simulink model "threelevel_12phase1"  (R2020b)
settings: Solver=FixedStepDiscrete  StartTime=0.0  StopTime=1  FixedStep=Ts_FEA  RelTol=1e-3
model workspace (MAT data in the model file):
  T_10kHz = Simulink.Parameter
  T_10kHz.DataType = 'auto'
  T_10kHz.Dimensions = [0 0]
undefined symbols (not defined in the file): Cin, DiscIntNeverNeededParam, ESL, ESR, faif, Jm, kfeed_r, ki_n, kp_n, L, Ld, Line, Lq, ncmd_climb, ncmd_cruise, ncmd_run, ncmd_takeoff, p, Pcmd_climb, Pcmd_cruise, Pcmd_run, Pcmd_takeoff, Rs, Tcmd_run, Tcmd_start, Tcmd_time, time_climb, time_cruise, time_run, time_start, time_takeoff, Ts, Ts_Dead, Ts_FEA, Ts_speedloop, tswitch_climb, tswitch_takeoff, VDC, ws, zero_C1
libraries: powerlib x73, simulink x16, powerlib_meascontrol x16, slpidlib x13
(part 1 of 6)
settings Model: SimulationMode=accelerator  Creator=Shaoy  LastModifiedBy=HP
settings SolverCC: MinimalZcImpactIntegration=on
settings DataIOCC: InitialState=xIntial  LoadInitialState=on  SaveFinalState=on  SaveOperatingPoint=on  SaveOutput=off  SignalLogging=off  DSMLogging=off  SaveTime=off  ReturnWorkspaceOutputs=off
settings DebuggingCC: ReadBeforeWriteMsg=DisableAll  WriteAfterWriteMsg=DisableAll  WriteAfterReadMsg=DisableAll  MultiTaskDSMMsg=none
settings ModelReferenceCC: UpdateModelReferenceTargets=IfOutOfDate
settings SFSimCC: SFSimEcho=off

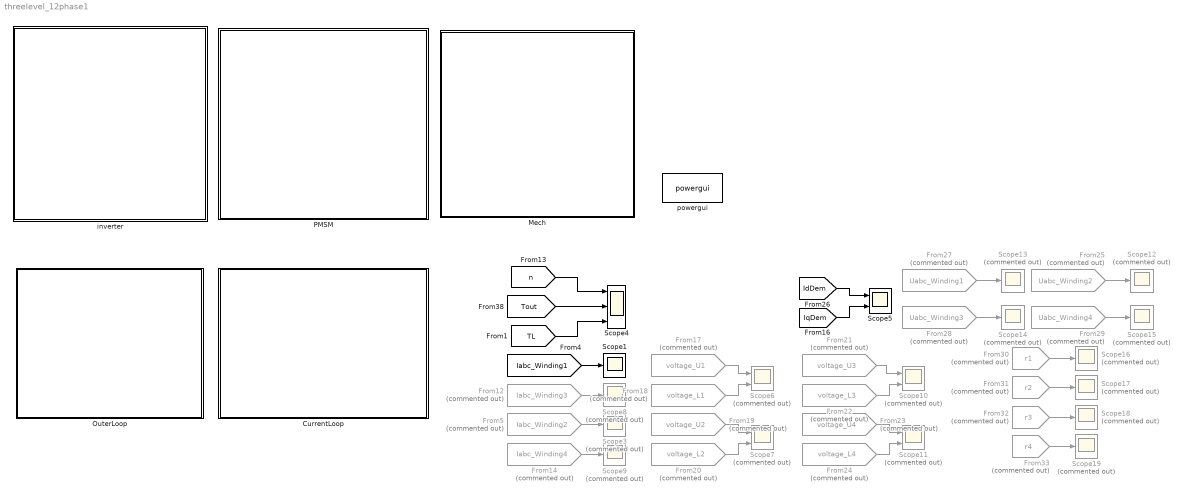
== system threelevel_12phase1 ==
  CurrentLoop : Subsystem
  From12 : From  Commented=on  GotoTag=Iabc_Winding3  TagVisibility=global
  From14 : From  Commented=on  GotoTag=Iabc_Winding4  TagVisibility=global
  From17 : From  Commented=on  GotoTag=voltage_U1  TagVisibility=global
  From18 : From  Commented=on  GotoTag=voltage_L1  TagVisibility=global
  From19 : From  Commented=on  GotoTag=voltage_U2  TagVisibility=global
  From20 : From  Commented=on  GotoTag=voltage_L2  TagVisibility=global
  From21 : From  Commented=on  GotoTag=voltage_U3  TagVisibility=global
  From22 : From  Commented=on  GotoTag=voltage_L3  TagVisibility=global
  From23 : From  Commented=on  GotoTag=voltage_U4  TagVisibility=global
  From24 : From  Commented=on  GotoTag=voltage_L4  TagVisibility=global
  From25 : From  Commented=on  GotoTag=Uabc_Winding2  TagVisibility=global
  From27 : From  Commented=on  GotoTag=Uabc_Winding1  TagVisibility=global
  From28 : From  Commented=on  GotoTag=Uabc_Winding3  TagVisibility=global
  From29 : From  Commented=on  GotoTag=Uabc_Winding4  TagVisibility=global
  From30 : From  Commented=on  GotoTag=r1  TagVisibility=global
  From31 : From  Commented=on  GotoTag=r2  TagVisibility=global
  From32 : From  Commented=on  GotoTag=r3  TagVisibility=global
  From33 : From  Commented=on  GotoTag=r4  TagVisibility=global
  From5 : From  Commented=on  GotoTag=Iabc_Winding2  TagVisibility=global
  Mech : Subsystem
  OuterLoop : Subsystem
  PMSM : Subsystem
  Scope1 : Scope
  Scope{6..7,10..11} (4 alike) : Scope  Commented=on  NumInputPorts=2
  Scope{3,8..9,12..19} (11 alike) : Scope  Commented=on
  Scope4 : Scope  NumInputPorts=3
  Scope5 : Scope  NumInputPorts=2
  inverter : Subsystem
  powergui : powerlib/powergui  Priority=1  SimulationMode=Discrete  SampleTime=Ts_FEA  frequency=60  Iterations=50  frequencyindice=0  Pbase=100e6  ErrMax=1e-4  UnitsV=kV  UnitsW=MW  buscounter=0  FunctionMessages=off  echomessages=off  EnableUseOfTLC=off  CurrentSourceSwitches=off  DisableSnubberDevices=off  DisableRonSwitches=off  DisableVfSwitches=off  DisplayEquations=off  AutomaticDiscreteSolvers=off  SolverType=Tustin/Backward Euler (TBE)  Interpol=off  ExternalGateDelay=off  methode=off  Ts=100  x0status=blocks  SPID=on  SwTol=0  HookPort=off  NonlinearTolerance=1e-4  nMaxIteration=100  ContinueOnMaxIteration=off  RestoreLinks=warning  ResistiveCurrentMeasurement=off  Frange=[0:2:500]  Ylog=off  Xlog=on  ShowGrid=off  save=off  variable=ZData  structure=Mech_out  ZoomFFT=off  StartTime=0.63  cycles=1  DisplayStyle=4  fundamental=6997*4/60  FreqAxis=off  MaxFrequency=100000  frequencyindicesteady=1  RmsSteady=1  display=off
  wires:
  [Iabc_Winding1] -> Scope1/1
  From5/1 -> Scope3/1
  From12/1 -> Scope8/1
  From14/1 -> Scope9/1
  [IqDem] -> Scope5/2
  From17/1 -> Scope6/1
  From18/1 -> Scope6/2
  From19/1 -> Scope7/1
  From20/1 -> Scope7/2
  From21/1 -> Scope10/1
  From22/1 -> Scope10/2
  From23/1 -> Scope11/1
  From24/1 -> Scope11/2
  From25/1 -> Scope12/1
  [IdDem] -> Scope5/1
  From27/1 -> Scope13/1
  From28/1 -> Scope14/1
  From29/1 -> Scope15/1
  From30/1 -> Scope16/1
  From31/1 -> Scope17/1
  From32/1 -> Scope18/1
  From33/1 -> Scope19/1
  [n] -> Scope4/1
  [Tout] -> Scope4/2
  [TL] -> Scope4/3

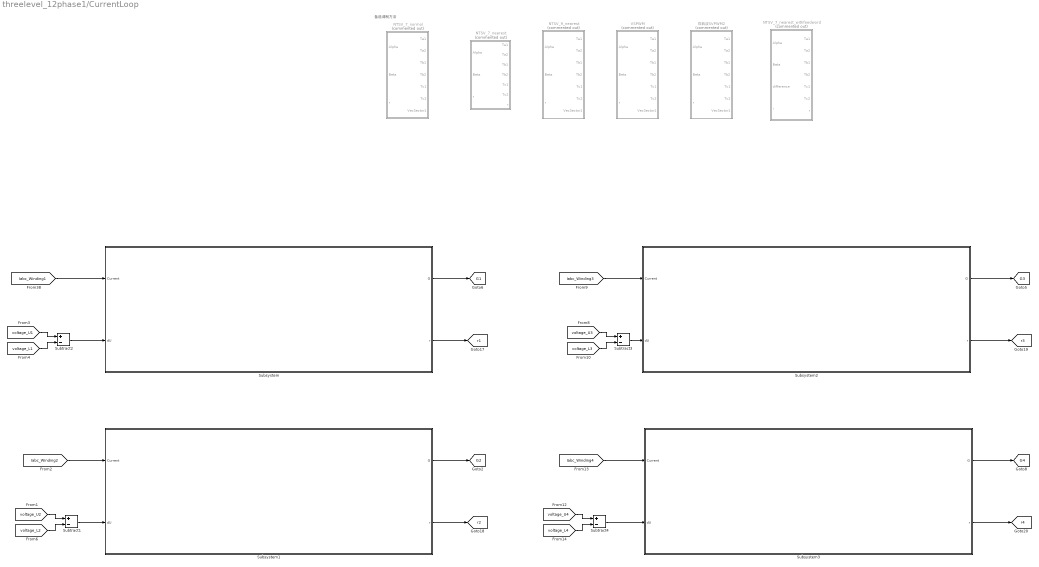
== system threelevel_12phase1/CurrentLoop ==
  note: 备选调制方法
  NTSV_7_nearest : MATLAB Function  Commented=on  TreatAsAtomicUnit=on
  NTSV_7_nearest_withfeedword : MATLAB Function  Commented=on  TreatAsAtomicUnit=on
  NTSV_7_normol : MATLAB Function  Commented=on  TreatAsAtomicUnit=on
  NTSV_9_nearest : MATLAB Function  Commented=on  TreatAsAtomicUnit=on
  Subsystem : Subsystem
  Subsystem1 : Subsystem
  Subsystem2 : Subsystem
  Subsystem3 : Subsystem
  Subtract{1..4} (4 alike) : Sum  Inputs=+-
  VSPWM : MATLAB Function  Commented=on  TreatAsAtomicUnit=on
  双载波SVPWM2 : MATLAB Function  Commented=on  TreatAsAtomicUnit=on
  tag scope: G1=global, G2=global, G3=global, G4=global, r1=global, r2=global, r3=global, r4=global
  wires:
  [voltage_U1] -> Subtract2/1
  [voltage_L1] -> Subtract2/2
  [voltage_L3] -> Subtract3/2
  [voltage_U3] -> Subtract3/1
  [voltage_L4] -> Subtract4/2
  [voltage_U4] -> Subtract4/1
  Subtract2/1 -> Subsystem/2(dU)
  [Iabc_Winding1] -> Subsystem/1(Current)
  Subsystem/2(r) -> [r1]
  Subsystem/1(G) -> [G1]
  Subtract1/1 -> Subsystem1/2(dU)
  [voltage_L2] -> Subtract1/2
  [voltage_U2] -> Subtract1/1
  [Iabc_Winding2] -> Subsystem1/1(Current)
  Subsystem1/2(r) -> [r2]
  Subsystem1/1(G) -> [G2]
  [Iabc_Winding3] -> Subsystem2/1(Current)
  Subtract3/1 -> Subsystem2/2(dU)
  Subsystem2/2(r) -> [r3]
  Subsystem2/1(G) -> [G3]
  Subsystem3/1(G) -> [G4]
  Subsystem3/2(r) -> [r4]
  [Iabc_Winding4] -> Subsystem3/1(Current)
  Subtract4/1 -> Subsystem3/2(dU)

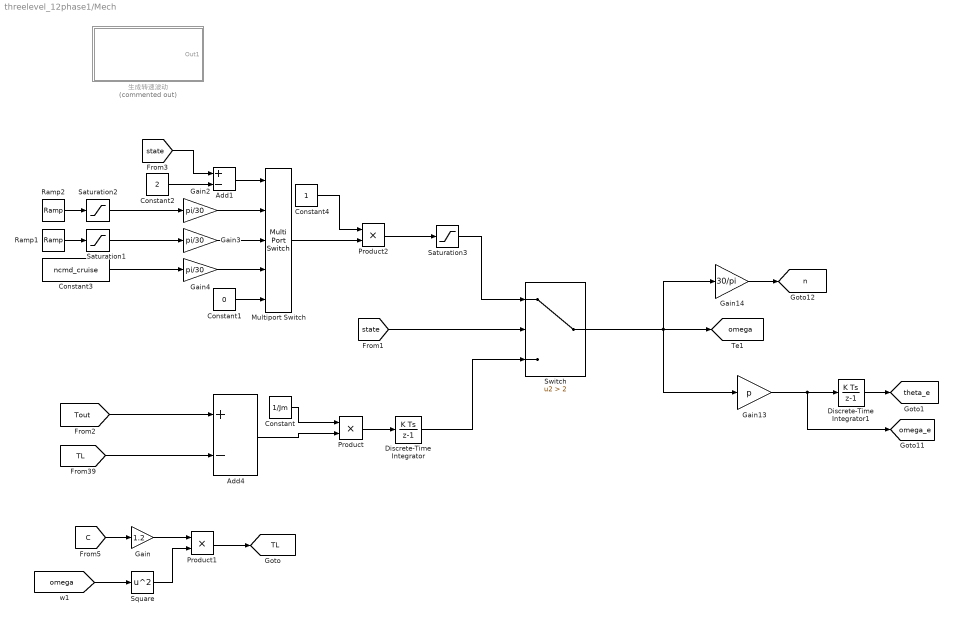
== system threelevel_12phase1/Mech ==
  Add1 : Sum  Inputs=+-
  Add4 : Sum  Inputs=+-
  Constant : Constant  Value=1/Jm  SampleTime=-1
  Constant1 : Constant  Value=0
  Constant2 : Constant  Value=2
  Constant3 : Constant  Value=ncmd_cruise
  Constant4 : Constant
  Discrete-Time Integrator : DiscreteIntegrator  SampleTime=-1  ICPrevOutput=DiscIntNeverNeededParam  ICPrevScaledInput=DiscIntNeverNeededParam
  Discrete-Time Integrator1 : DiscreteIntegrator  SampleTime=-1  ICPrevOutput=DiscIntNeverNeededParam  ICPrevScaledInput=DiscIntNeverNeededParam
  Gain : Gain  Gain=1.2
  Gain13 : Gain  Gain=p
  Gain14 : Gain  Gain=30/pi
  Gain2 : Gain  Gain=pi/30
  Gain3 : Gain  Gain=pi/30
  Gain4 : Gain  Gain=pi/30
  Multiport Switch : MultiPortSwitch  DataPortForDefault=Additional data port  DiagnosticForDefault=None
  Product : Product
  Product1 : Product
  Product2 : Product
  Ramp1 : simulink/Sources/Ramp  slope=(ncmd_climb-ncmd_takeoff)/tswitch_climb  start=time_takeoff  InitialOutput=ncmd_takeoff
  Ramp2 : simulink/Sources/Ramp  slope=(ncmd_takeoff-ncmd_run)/tswitch_takeoff  start=time_run  InitialOutput=ncmd_run
  Saturation1 : Saturate  UpperLimit=ncmd_takeoff  LowerLimit=ncmd_climb
  Saturation2 : Saturate  UpperLimit=ncmd_takeoff  LowerLimit=ncmd_run
  Saturation3 : Saturate  UpperLimit=988  LowerLimit=0
  Square : Math  Operator=square  SaturateOnIntegerOverflow=on
  Switch : Switch  Criteria=u2 > Threshold  Threshold=2
  生成转速波动 : Subsystem  Commented=on
  tag scope: TL=global, n=global, omega=global, omega_e=global, theta_e=global
  wires:
  [Tout] -> Add4/1
  Add4/1 -> Product/2
  Product/1 -> Discrete-Time Integrator/1
  Constant/1 -> Product/1
  [TL] -> Add4/2
  Gain14/1 -> [n]
  [C] -> Gain/1
  Gain/1 -> Product1/1
  Product1/1 -> [TL]
  [omega] -> Square/1
  Square/1 -> Product1/2
  Discrete-Time Integrator1/1 -> [theta_e]
  Gain13/1 -> [omega_e], Discrete-Time Integrator1/1
  Switch/1 -> Gain14/1, Gain13/1, [omega]
  [state] -> Switch/2
  Discrete-Time Integrator/1 -> Switch/3
  Constant1/1 -> Multiport Switch/5
  [state] -> Add1/1
  Add1/1 -> Multiport Switch/1
  Constant2/1 -> Add1/2
  Gain4/1 -> Multiport Switch/4
  Gain3/1 -> Multiport Switch/3
  Gain2/1 -> Multiport Switch/2
  Saturation2/1 -> Gain2/1
  Saturation1/1 -> Gain3/1
  Constant3/1 -> Gain4/1
  Ramp2/1 -> Saturation2/1
  Ramp1/1 -> Saturation1/1
  Multiport Switch/1 -> Product2/2
  Product2/1 -> Saturation3/1
  Saturation3/1 -> Switch/1
  Constant4/1 -> Product2/1

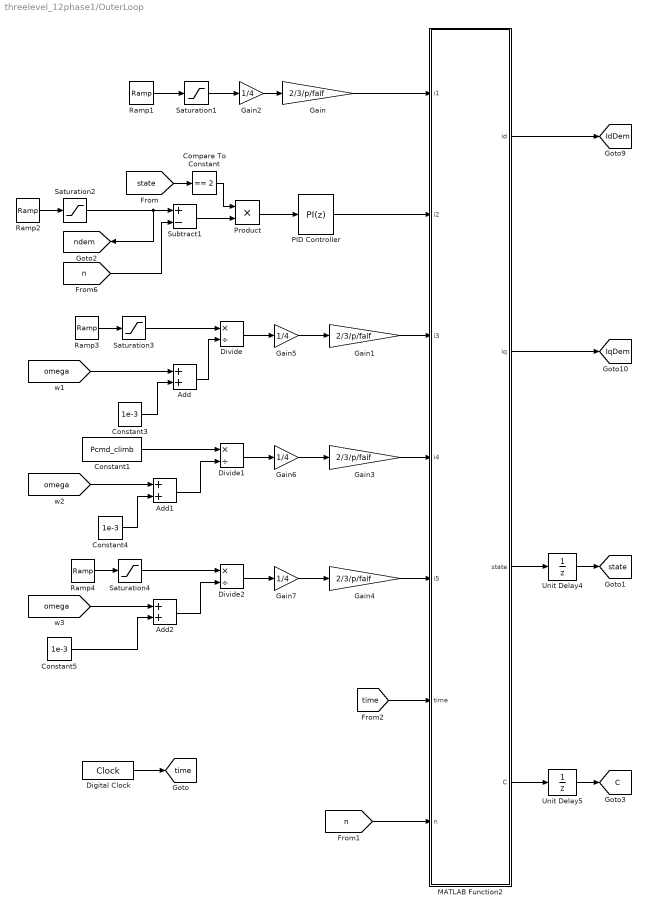
== system threelevel_12phase1/OuterLoop ==
  Add : Sum
  Add1 : Sum
  Add2 : Sum
  Compare To Constant : simulink/Logic and Bit Operations/Compare To Constant  relop===  const=2  OutDataTypeStr=boolean
  Constant1 : Constant  Value=Pcmd_climb
  Constant3 : Constant  Value=1e-3
  Constant4 : Constant  Value=1e-3
  Constant5 : Constant  Value=1e-3
  Digital Clock : DigitalClock
  Divide : Product  Inputs=*/
  Divide1 : Product  Inputs=*/
  Divide2 : Product  Inputs=*/
  Gain{,1,3..4} (4 alike) : Gain  Gain=2/3/p/faif
  Gain{2,5..7} (4 alike) : Gain  Gain=1/4
  MATLAB Function2 : MATLAB Function  TreatAsAtomicUnit=on
  PID Controller : slpidlib/PID Controller  Controller=PI  Form=Parallel  TimeDomain=Discrete-time  UseExternalTs=off  SampleTime=Ts_speedloop  IntegratorMethod=Forward Euler  FilterMethod=Forward Euler  ControllerParametersSource=internal  P=kp_n  I=ki_n  D=0  UseFilter=on  N=100  TunerSelectOption=Transfer Function Based (PID Tuner App)  InitialConditionSource=internal  InitialConditionForIntegrator=2*Tcmd_run/4/3/p/faif  InitialConditionForFilter=0  DifferentiatorICPrevScaledInput=0  ExternalReset=none  TrackingMode=off  Kt=1  LimitOutput=off  SatLimitsSource=internal  UpperSaturationLimit=1  LowerSaturationLimit=-1  LinearizeAsGain=off  AntiWindupMode=none  Kb=1  POutMin=[]  POutMax=[]  IOutMin=[]  IOutMax=[]  DOutMin=[]  DOutMax=[]  NOutMin=[]  NOutMax=[]  SumOutMin=[]  SumOutMax=[]  SaturationOutMin=[]  SaturationOutMax=[]  PParamMin=[]  PParamMax=[]  IParamMin=[]  IParamMax=[]  DParamMin=[]  DParamMax=[]  NParamMin=[]  NParamMax=[]  KbParamMin=[]  KbParamMax=[]  KtParamMin=[]  KtParamMax=[]  KbOutMin=[]  KbOutMax=[]  KtOutMin=[]  KtOutMax=[]  IntegratorOutMin=[]  IntegratorOutMax=[]  FilterOutMin=[]  FilterOutMax=[]  SumI1OutMin=[]  SumI1OutMax=[]  SumI2OutMin=[]  SumI2OutMax=[]  SumI3OutMin=[]  SumI3OutMax=[]  SumI4OutMin=[]  SumI4OutMax=[]  SumDOutMin=[]  SumDOutMax=[]  DifferentiatorOutMin=[]  DifferentiatorOutMax=[]  FilterDiffOutCoefMin=[]  FilterDiffOutCoefMax=[]  ReciprocalOutMin=[]  ReciprocalOutMax=[]  SumDenOutMin=[]  SumDenOutMax=[]  SumNumOutMin=[]  SumNumOutMax=[]  DivideOutMin=[]  DivideOutMax=[]  UdiffTsProdOutMin=[]  UdiffTsProdOutMax=[]  NTsProdOutMin=[]  NTsProdOutMax=[]  UintegralTsProdOutMin=[]  UintegralTsProdOutMax=[]  UngainTsProdOutMin=[]  UngainTsProdOutMax=[]  IntegratorContinuousStateAttributes=''  IntegratorStateMustResolveToSignalObject=off  IntegratorRTWStateStorageClass=Auto  FilterContinuousStateAttributes=''  FilterStateMustResolveToSignalObject=off  FilterRTWStateStorageClass=Auto  ParallelPVariant=InternalParameters  IdealPVariant=Disabled  IVariant=InternalParameters  DVariant=Disabled  IntegratorVariant=Discrete  SatVariant=Disabled  AWVariant=Passthrough  PCopyVariant=Disabled  TRVariant=Disabled  FdbkBlocksVariant=Forward  IdealPFdbkVariant=Disabled  SatFdbkVariant=Disabled  DerivativeFilterVariant=Disabled  NVariant=Disabled  NCopyVariant=Disabled_SignalSpec  FilterICVariant=Disabled  IntegratorICVariant=InternalICs  ExternalResetVariant=Disabled  TRSumVariant=Passthrough  SumFdbkVariant=Disabled  SumVariant=Sum_PI  TsampFilterVariant=InternalTs  TsampNgainVariant=Passthrough  TsampIntegralVariant=Passthrough  ExternalSaturationOutDataTypeStr=Inherit: Same as second input
  Product : Product
  Ramp1 : simulink/Sources/Ramp  slope=Tcmd_start/Tcmd_time  start=0  InitialOutput=0
  Ramp2 : simulink/Sources/Ramp  slope=ncmd_run/0.1  start=0  InitialOutput=0
  Ramp3 : simulink/Sources/Ramp  slope=(Pcmd_takeoff-Pcmd_run)/tswitch_climb  start=time_run  InitialOutput=Pcmd_run
  Ramp4 : simulink/Sources/Ramp  slope=(Pcmd_cruise-Pcmd_climb)/tswitch_climb  start=time_climb  InitialOutput=Pcmd_climb
  Saturation1 : Saturate  UpperLimit=Tcmd_start  LowerLimit=0
  Saturation2 : Saturate  UpperLimit=ncmd_run  LowerLimit=0
  Saturation3 : Saturate  UpperLimit=Pcmd_takeoff  LowerLimit=0
  Saturation4 : Saturate  UpperLimit=Pcmd_takeoff  LowerLimit=Pcmd_cruise
  Subtract1 : Sum  Inputs=+-
  Unit Delay4 : UnitDelay  SampleTime=-1  HasFrameUpgradeWarning=on
  Unit Delay5 : UnitDelay  SampleTime=-1  HasFrameUpgradeWarning=on
  tag scope: C=global, IdDem=global, IqDem=global, ndem=global, state=global, time=global
  wires:
  Saturation1/1 -> Gain2/1
  Ramp1/1 -> Saturation1/1
  Gain2/1 -> Gain/1
  Saturation2/1 -> [ndem], Subtract1/1
  Ramp2/1 -> Saturation2/1
  Subtract1/1 -> Product/2
  Product/1 -> PID Controller/1
  Gain/1 -> MATLAB Function2/1(i1)
  PID Controller/1 -> MATLAB Function2/2(i2)
  Gain1/1 -> MATLAB Function2/3(i3)
  Add1/1 -> Divide1/2
  Constant1/1 -> Divide1/1
  Saturation4/1 -> Divide2/1
  Add2/1 -> Divide2/2
  MATLAB Function2/3(state) -> Unit Delay4/1
  MATLAB Function2/4(C) -> Unit Delay5/1
  [state] -> Compare To Constant/1
  Compare To Constant/1 -> Product/1
  MATLAB Function2/1(id) -> [IdDem]
  MATLAB Function2/2(iq) -> [IqDem]
  Constant3/1 -> Add/2
  Add/1 -> Divide/2
  Constant4/1 -> Add1/2
  Constant5/1 -> Add2/2
  Gain3/1 -> MATLAB Function2/4(i4)
  Gain4/1 -> MATLAB Function2/5(i5)
  [n] -> MATLAB Function2/7(n)
  [omega] -> Add/1
  [omega] -> Add1/1
  [omega] -> Add2/1
  Ramp3/1 -> Saturation3/1
  Saturation3/1 -> Divide/1
  Gain7/1 -> Gain4/1
  Divide2/1 -> Gain7/1
  Divide1/1 -> Gain6/1
  Gain6/1 -> Gain3/1
  Gain5/1 -> Gain1/1
  Divide/1 -> Gain5/1
  [n] -> Subtract1/2
  Unit Delay4/1 -> [state]
  Unit Delay5/1 -> [C]
  Ramp4/1 -> Saturation4/1
  [time] -> MATLAB Function2/6(time)
  Digital Clock/1 -> [time]

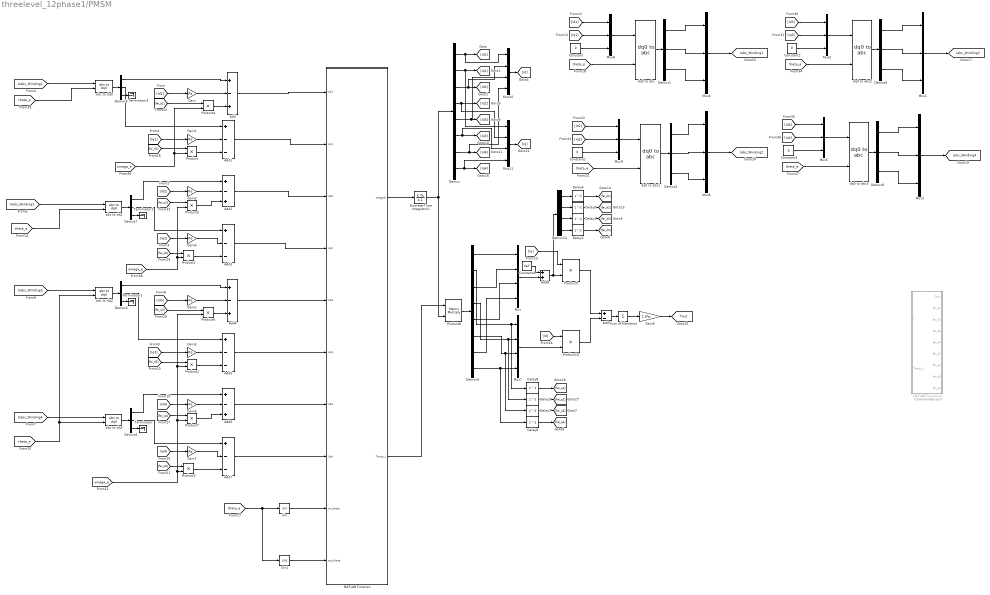
== system threelevel_12phase1/PMSM ==
  Add{,2,4,6} (4 alike) : Sum  Inputs=+-+
  Add{1,3,5,7} (4 alike) : Sum  Inputs=+--
  Add8 : Sum
  Add9 : Sum  Inputs=+-
  Constant{,1..3} (4 alike) : Constant  Value=0  SampleTime=-1
  Constant4 : Constant  Value=faif
  Delay{1..6,8..9} (8 alike) : Delay  DelayLength=1
  Demux : Demux  Outputs=8
  Demux{1..8} (8 alike) : Demux  Outputs=3
  Demux10 : Demux
  Demux9 : Demux  Outputs=8
  Discrete-Time Integrator1 : DiscreteIntegrator  SampleTime=-1  ICPrevOutput=DiscIntNeverNeededParam  ICPrevScaledInput=DiscIntNeverNeededParam
  Gain{,1..7} (8 alike) : Gain  Gain=Rs
  Gain8 : Gain  Gain=1.5*p
  MATLAB Function : MATLAB Function  TreatAsAtomicUnit=on
  MATLAB Function2 : MATLAB Function  Commented=on  TreatAsAtomicUnit=on
  Mux{,7,10..11} (4 alike) : Mux
  Mux{1..6,8..9} (8 alike) : Mux  Inputs=3
  Product{,1..7,9..10} (10 alike) : Product
  Product8 : Product  Multiplication=Matrix(*)
  Sin : Trigonometry
  Sin1 : Trigonometry  Operator=cos
  Sum of Elements : Sum  Inputs=+
  Terminator{,1..3} (4 alike) : Terminator
  abc to dq{0..3} (4 alike) : powerlib_meascontrol/Transformations/abc to dq0  Alignment=Aligned with phase A axis
  dq0 to abc{,1..3} (4 alike) : powerlib_meascontrol/Transformations/dq0 to abc  Alignment=Aligned with phase A axis
  tag scope: Iabc_Winding1=global, Iabc_Winding2=global, Iabc_Winding3=global, Iabc_Winding4=global, Tout=global
  wires:
  Demux5/2 -> Add1/1
  Demux5/1 -> Add/1
  Gain/1 -> Add/2
  [Id1] -> Gain/1
  [Iq1] -> Gain1/1
  Gain1/1 -> Add1/2
  Gain4/1 -> Add3/2
  [Iq2] -> Gain4/1
  [Id2] -> Gain3/1
  Gain3/1 -> Add2/2
  Demux7/1 -> Add2/1
  Demux7/2 -> Add3/1
  Add/1 -> MATLAB Function/1(Ud1)
  Add1/1 -> MATLAB Function/2(Uq1)
  [Uabc_Winding2] -> abc to dq1/1
  [Id1] -> Mux8/1
  [Iq1] -> Mux8/2
  Constant/1 -> Mux8/3
  [theta_e] -> abc to dq1/2
  [theta_e] -> dq0 to abc/2
  Demux1/1 -> Mux4/1
  Demux1/2 -> Mux4/2
  Demux1/3 -> Mux4/3
  Demux2/3 -> Mux6/3
  Demux2/2 -> Mux6/2
  Demux2/1 -> Mux6/1
  [theta_e] -> dq0 to abc1/2
  [Iq2] -> Mux9/2
  [Id2] -> Mux9/1
  Mux4/1 -> [Iabc_Winding1]
  Mux6/1 -> [Iabc_Winding2]
  Add2/1 -> MATLAB Function/3(Ud2)
  Add3/1 -> MATLAB Function/4(Uq2)
  abc to dq0/1 -> Demux5/1
  abc to dq1/1 -> Demux7/1
  Mux8/1 -> dq0 to abc/1
  dq0 to abc/1 -> Demux1/1
  dq0 to abc1/1 -> Demux2/1
  Mux9/1 -> dq0 to abc1/1
  Discrete-Time Integrator1/1 -> Product8/2, Demux/1
  [Uabc_Winding1] -> abc to dq0/1
  MATLAB Function/1(Integral) -> Discrete-Time Integrator1/1
  Demux/1 -> Mux10/1, [Id1]
  Demux/2 -> Mux11/1, [Iq1]
  Demux/3 -> Mux10/2, [Id2]
  Demux/4 -> Mux11/2, [Iq2]
  Constant1/1 -> Mux9/3
  Delay4/1 -> [fai_d1]
  Delay5/1 -> [fai_d2]
  Delay8/1 -> [fai_q1]
  Delay9/1 -> [fai_q2]
  Product/1 -> Add1/3
  [fai_d1] -> Product/1
  Product1/1 -> Add3/3
  [fai_d2] -> Product1/1
  Product4/1 -> Add/3
  [fai_q1] -> Product4/1
  Product5/1 -> Add2/3
  [fai_q2] -> Product5/1
  [Uabc_Winding4] -> abc to dq3/1
  [theta_e] -> abc to dq3/2, abc to dq2/2
  [Id3] -> Gain2/1
  Demux4/2 -> Add7/1
  Gain2/1 -> Add4/2
  Gain6/1 -> Add6/2
  [Iq4] -> Gain7/1
  Gain7/1 -> Add7/2
  Demux3/1 -> Add4/1
  [omega_e] -> Product7/2, Product6/2, Product2/2, Product3/2
  [Iq3] -> Gain5/1
  [fai_d3] -> Product2/1
  Demux4/1 -> Add6/1
  Product6/1 -> Add4/3
  Product7/1 -> Add6/3
  [fai_d4] -> Product3/1
  [fai_q4] -> Product7/1
  Product3/1 -> Add7/3
  Gain5/1 -> Add5/2
  Product2/1 -> Add5/3
  Demux3/2 -> Add5/1
  [Id4] -> Gain6/1
  [Uabc_Winding3] -> abc to dq2/1
  abc to dq2/1 -> Demux3/1
  [fai_q3] -> Product6/1
  abc to dq3/1 -> Demux4/1
  Add4/1 -> MATLAB Function/5(Ud3)
  Add5/1 -> MATLAB Function/6(Uq3)
  Add6/1 -> MATLAB Function/7(Ud4)
  Add7/1 -> MATLAB Function/8(Uq4)
  Delay1/1 -> [fai_d3]
  Delay2/1 -> [fai_d4]
  Delay6/1 -> [fai_q4]
  Delay3/1 -> [fai_q3]
  Demux/5 -> Mux10/3, [Id3]
  Demux/6 -> Mux11/3, [Iq3]
  Demux/7 -> Mux10/4, [Id4]
  Demux/8 -> Mux11/4, [Iq4]
  Mux1/1 -> [Iabc_Winding3]
  Mux2/1 -> dq0 to abc2/1
  Demux6/2 -> Mux1/2
  Constant2/1 -> Mux2/3
  dq0 to abc2/1 -> Demux6/1
  [Id3] -> Mux2/1
  [theta_e] -> dq0 to abc2/2
  Demux6/3 -> Mux1/3
  Demux6/1 -> Mux1/1
  [Iq3] -> Mux2/2
  Mux3/1 -> [Iabc_Winding4]
  Demux8/2 -> Mux3/2
  dq0 to abc3/1 -> Demux8/1
  Constant3/1 -> Mux5/3
  [theta_e] -> dq0 to abc3/2
  [Id4] -> Mux5/1
  [Iq4] -> Mux5/2
  Mux5/1 -> dq0 to abc3/1
  Demux8/3 -> Mux3/3
  Demux8/1 -> Mux3/1
  Demux4/3 -> Terminator/1
  Demux3/3 -> Terminator1/1
  Demux7/3 -> Terminator2/1
  Demux5/3 -> Terminator3/1
  [theta_e] -> Sin1/1, Sin/1
  Sin/1 -> MATLAB Function/9(sin_theta)
  Sin1/1 -> MATLAB Function/10(cos_theta)
  MATLAB Function/2(Temp_L) -> Product8/1
  Product8/1 -> Demux9/1
  Demux9/1 -> Mux/1
  Demux9/3 -> Mux/2
  Demux9/5 -> Mux/3
  Demux9/7 -> Mux/4
  Mux/1 -> Add8/2
  Constant4/1 -> Add8/1
  Demux9/8 -> Delay6/1, Mux7/4
  Demux9/6 -> Mux7/3, Delay3/1
  Demux9/2 -> Delay8/1, Mux7/1
  Demux9/4 -> Delay9/1, Mux7/2
  Mux10/1 -> [Id]
  Mux11/1 -> [Iq]
  Add8/1 -> Demux10/1, Product9/2
  [Iq] -> Product9/1
  Mux7/1 -> Product10/2
  [Id] -> Product10/1
  Product9/1 -> Add9/1
  Product10/1 -> Add9/2
  Add9/1 -> Sum of Elements/1
  Sum of Elements/1 -> Gain8/1
  Gain8/1 -> [Tout]
  Demux10/1 -> Delay4/1
  Demux10/2 -> Delay5/1
  Demux10/3 -> Delay1/1
  Demux10/4 -> Delay2/1
  [theta_e] -> abc to dq0/2
  [omega_e] -> Product5/2, Product1/2
  [omega_e] -> Product4/2, Product/2

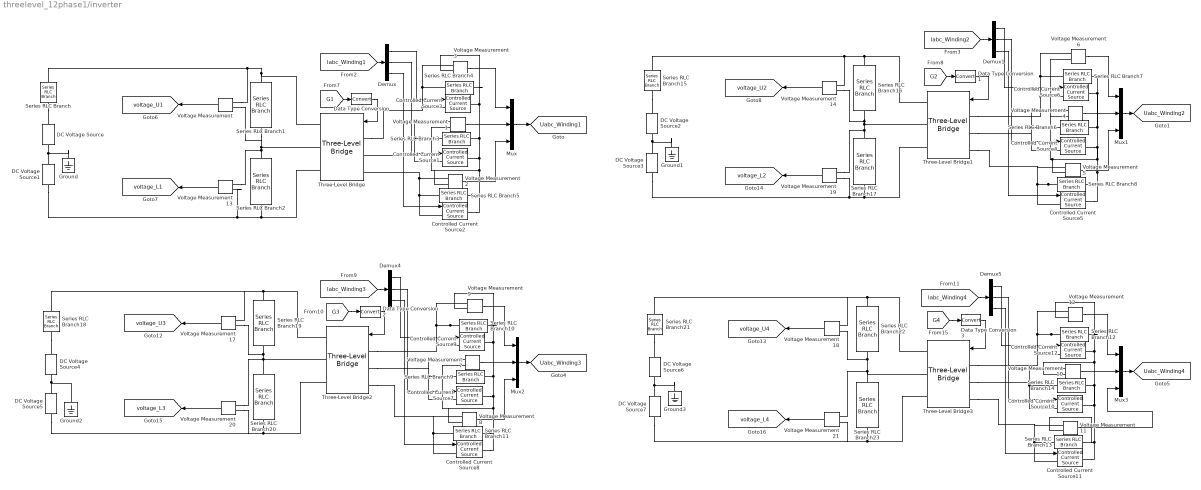
== system threelevel_12phase1/inverter ==
  Controlled Current Source{1..12} (12 alike) : powerlib/Electrical Sources/Controlled Current Source  Initialize=on  Source_Type=AC  Amplitude=0  Phase=0  Frequency=0  Measurements=None
  DC Voltage Source{,1..7} (8 alike) : powerlib/Electrical Sources/DC Voltage Source  Amplitude=VDC/2  Measurements=None
  Data Type Conversion{,1..3} (4 alike) : DataTypeConversion
  Demux{,1,4..5} (4 alike) : Demux  Outputs=3
  Ground{,1..3} (4 alike) : powerlib/Elements/Ground  LConnTagsString=a
  Mux{,1..3} (4 alike) : Mux  Inputs=3
  Series RLC Branch{,15,18,21} (4 alike) : powerlib/Elements/Series RLC Branch  LConnTagsString=__new0  RConnTagsString=__new0  BranchType=L  Resistance=1  Inductance=Line  SetiL0=off  InitialCurrent=0  Capacitance=1e-6  Setx0=off  InitialVoltage=0  Measurements=None
  Series RLC Branch{1..2,16..17,19..20,22..23} (8 alike) : powerlib/Elements/Series RLC Branch  LConnTagsString=__new0  RConnTagsString=__new0  BranchType=RLC  Resistance=ESR  Inductance=ESL  SetiL0=off  InitialCurrent=0  Capacitance=Cin  Setx0=off  InitialVoltage=0  Measurements=None
  Series RLC Branch{3..14} (12 alike) : powerlib/Elements/Series RLC Branch  LConnTagsString=__new0  RConnTagsString=__new0  BranchType=R  Resistance=10^6  Inductance=51.869e-9  SetiL0=off  InitialCurrent=0  Capacitance=330e-6  Setx0=off  InitialVoltage=0  Measurements=None
  Three-Level Bridge{,1..3} (4 alike) : powerlib/Power Electronics/Three-Level Bridge  Arms=3  SnubberResistance=1e5  SbubberCapacitance=inf  Device=IGBT / Diodes  Ron=3.1e-3  ForwardVoltages="[  0.77  0.9  ]"  Measurements=None
      settings: SourceProductBaseCode=PS
  Voltage Measurement{,1..14,17..21} (20 alike) : powerlib/Measurements/Voltage Measurement  PhasorSimulation=off  OutputType=Complex  PSBequivalent=0
  tag scope: Uabc_Winding1=global, Uabc_Winding2=global, Uabc_Winding3=global, Uabc_Winding4=global, voltage_L1=global, voltage_L2=global, voltage_L3=global, voltage_L4=global, voltage_U1=global, voltage_U2=global, voltage_U3=global, voltage_U4=global
  wires:
  [G4] -> Data Type Conversion3/1
  Demux5/3 -> Controlled Current Source11/1
  Voltage Measurement9/1 -> Mux2/1
  Mux/1 -> [Uabc_Winding1]
  [Iabc_Winding3] -> Demux4/1
  Demux/3 -> Controlled Current Source2/1
  Demux/1 -> Controlled Current Source3/1
  [Iabc_Winding1] -> Demux/1
  Voltage Measurement3/1 -> Mux/1
  Voltage Measurement2/1 -> Mux/3
  Voltage Measurement6/1 -> Mux1/1
  Demux1/1 -> Controlled Current Source6/1
  Voltage Measurement21/1 -> [voltage_L4]
  Mux1/1 -> [Uabc_Winding2]
  Demux1/3 -> Controlled Current Source5/1
  Demux4/1 -> Controlled Current Source9/1
  [G3] -> Data Type Conversion2/1
  Demux4/3 -> Controlled Current Source8/1
  Voltage Measurement7/1 -> Mux2/2
  Demux4/2 -> Controlled Current Source7/1
  Data Type Conversion2/1 -> Three-Level Bridge2/1
  Voltage Measurement8/1 -> Mux2/3
  Voltage Measurement/1 -> [voltage_U1]
  Voltage Measurement4/1 -> Mux1/2
  Demux/2 -> Controlled Current Source1/1
  Voltage Measurement17/1 -> [voltage_U3]
  Mux2/1 -> [Uabc_Winding3]
  Voltage Measurement10/1 -> Mux3/2
  Demux5/1 -> Controlled Current Source12/1
  Voltage Measurement19/1 -> [voltage_L2]
  Mux3/1 -> [Uabc_Winding4]
  [G2] -> Data Type Conversion1/1
  [Iabc_Winding4] -> Demux5/1
  Voltage Measurement13/1 -> [voltage_L1]
  Voltage Measurement11/1 -> Mux3/3
  Voltage Measurement12/1 -> Mux3/1
  Voltage Measurement20/1 -> [voltage_L3]
  [G1] -> Data Type Conversion/1
  Voltage Measurement1/1 -> Mux/2
  Demux1/2 -> Controlled Current Source4/1
  Voltage Measurement18/1 -> [voltage_U4]
  Data Type Conversion/1 -> Three-Level Bridge/1
  Voltage Measurement5/1 -> Mux1/3
  Voltage Measurement14/1 -> [voltage_U2]
  [Iabc_Winding2] -> Demux1/1
  Data Type Conversion1/1 -> Three-Level Bridge1/1
  Data Type Conversion3/1 -> Three-Level Bridge3/1
  Demux5/2 -> Controlled Current Source10/1
  connections:
  Voltage Measurement10/LConn1 -- Three-Level Bridge3/LConn2 -- Controlled Current Source10/LConn1 -- Series RLC Branch14/LConn1
  Series RLC Branch19/RConn1 -- Voltage Measurement17/LConn2 -- Series RLC Branch20/LConn1 -- Three-Level Bridge2/RConn2 -- Voltage Measurement20/LConn1
  Controlled Current Source7/RConn1 -- Voltage Measurement7/LConn2 -- Voltage Measurement8/LConn2 -- Controlled Current Source8/RConn1 -- Series RLC Branch11/RConn1 -- Voltage Measurement9/LConn2 -- Series RLC Branch10/RConn1 -- Controlled Current Source9/RConn1 -- Series RLC Branch9/RConn1
  Series RLC Branch5/RConn1 -- Controlled Current Source2/RConn1 -- Voltage Measurement1/LConn2 -- Voltage Measurement2/LConn2 -- Controlled Current Source1/RConn1 -- Voltage Measurement3/LConn2 -- Series RLC Branch4/RConn1 -- Controlled Current Source3/RConn1 -- Series RLC Branch3/RConn1
  Controlled Current Source6/LConn1 -- Three-Level Bridge1/LConn1 -- Voltage Measurement6/LConn1 -- Series RLC Branch7/LConn1
  DC Voltage Source1/LConn1 -- Voltage Measurement13/LConn2 -- Three-Level Bridge/RConn3 -- Series RLC Branch2/RConn1
  Controlled Current Source11/LConn1 -- Three-Level Bridge3/LConn3 -- Voltage Measurement11/LConn1 -- Series RLC Branch13/LConn1
  Controlled Current Source10/RConn1 -- Voltage Measurement11/LConn2 -- Series RLC Branch13/RConn1 -- Controlled Current Source11/RConn1 -- Voltage Measurement10/LConn2 -- Voltage Measurement12/LConn2 -- Series RLC Branch12/RConn1 -- Controlled Current Source12/RConn1 -- Series RLC Branch14/RConn1
  Controlled Current Source3/LConn1 -- Three-Level Bridge/LConn1 -- Voltage Measurement3/LConn1 -- Series RLC Branch4/LConn1
  Series RLC Branch18/LConn1 -- Voltage Measurement17/LConn1 -- Three-Level Bridge2/RConn1 -- Series RLC Branch19/LConn1
  DC Voltage Source1/RConn1 -- Ground/LConn1 -- DC Voltage Source/LConn1
  Series RLC Branch10/LConn1 -- Voltage Measurement9/LConn1 -- Three-Level Bridge2/LConn1 -- Controlled Current Source9/LConn1
  Voltage Measurement4/LConn1 -- Three-Level Bridge1/LConn2 -- Controlled Current Source4/LConn1 -- Series RLC Branch6/LConn1
  Series RLC Branch8/LConn1 -- Three-Level Bridge1/LConn3 -- Voltage Measurement5/LConn1 -- Controlled Current Source5/LConn1
  Series RLC Branch12/LConn1 -- Three-Level Bridge3/LConn1 -- Controlled Current Source12/LConn1 -- Voltage Measurement12/LConn1
  Series RLC Branch22/RConn1 -- Voltage Measurement18/LConn2 -- Three-Level Bridge3/RConn2 -- Series RLC Branch23/LConn1 -- Voltage Measurement21/LConn1
  Three-Level Bridge2/LConn2 -- Voltage Measurement7/LConn1 -- Controlled Current Source7/LConn1 -- Series RLC Branch9/LConn1
  Controlled Current Source1/LConn1 -- Three-Level Bridge/LConn2 -- Voltage Measurement1/LConn1 -- Series RLC Branch3/LConn1
  Controlled Current Source8/LConn1 -- Three-Level Bridge2/LConn3 -- Voltage Measurement8/LConn1 -- Series RLC Branch11/LConn1
  Series RLC Branch7/RConn1 -- Voltage Measurement6/LConn2 -- Voltage Measurement4/LConn2 -- Voltage Measurement5/LConn2 -- Series RLC Branch8/RConn1 -- Controlled Current Source5/RConn1 -- Controlled Current Source4/RConn1 -- Series RLC Branch6/RConn1 -- Controlled Current Source6/RConn1
  Series RLC Branch16/RConn1 -- Voltage Measurement14/LConn2 -- Three-Level Bridge1/RConn2 -- Voltage Measurement19/LConn1 -- Series RLC Branch17/LConn1
  Voltage Measurement2/LConn1 -- Controlled Current Source2/LConn1 -- Series RLC Branch5/LConn1 -- Three-Level Bridge/LConn3
  Voltage Measurement13/LConn1 -- Series RLC Branch1/RConn1 -- Voltage Measurement/LConn2 -- Three-Level Bridge/RConn2 -- Series RLC Branch2/LConn1
  Series RLC Branch/RConn1 -- DC Voltage Source/RConn1
  DC Voltage Source7/LConn1 -- Voltage Measurement21/LConn2 -- Three-Level Bridge3/RConn3 -- Series RLC Branch23/RConn1
  Voltage Measurement19/LConn2 -- Three-Level Bridge1/RConn3 -- Series RLC Branch17/RConn1 -- DC Voltage Source3/LConn1
  DC Voltage Source5/LConn1 -- Voltage Measurement20/LConn2 -- Three-Level Bridge2/RConn3 -- Series RLC Branch20/RConn1
  DC Voltage Source2/LConn1 -- DC Voltage Source3/RConn1 -- Ground1/LConn1
  Series RLC Branch15/RConn1 -- DC Voltage Source2/RConn1
  Voltage Measurement/LConn1 -- Series RLC Branch/LConn1 -- Three-Level Bridge/RConn1 -- Series RLC Branch1/LConn1
  Series RLC Branch16/LConn1 -- Three-Level Bridge1/RConn1 -- Voltage Measurement14/LConn1 -- Series RLC Branch15/LConn1
  Voltage Measurement18/LConn1 -- Series RLC Branch21/LConn1 -- Three-Level Bridge3/RConn1 -- Series RLC Branch22/LConn1
  DC Voltage Source4/LConn1 -- DC Voltage Source5/RConn1 -- Ground2/LConn1
  Series RLC Branch18/RConn1 -- DC Voltage Source4/RConn1
  DC Voltage Source6/LConn1 -- DC Voltage Source7/RConn1 -- Ground3/LConn1
  Series RLC Branch21/RConn1 -- DC Voltage Source6/RConn1

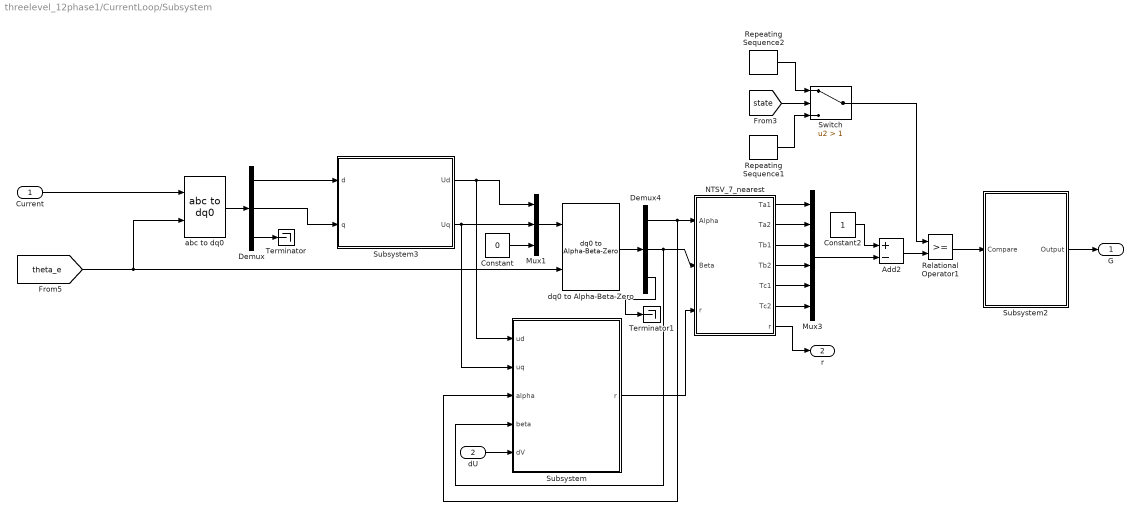
== system threelevel_12phase1/CurrentLoop/Subsystem ==
  Current : Inport
  dU : Inport  Port=2
  Add2 : Sum  Inputs=+-  AccumDataTypeStr=double  OutDataTypeStr=double
  Constant : Constant  Value=0
  Constant2 : Constant  OutDataTypeStr=double
  Demux : Demux  Outputs=3
  Demux4 : Demux  Outputs=3
  Mux1 : Mux  Inputs=3
  Mux3 : Mux  Inputs=6
  NTSV_7_nearest : MATLAB Function  TreatAsAtomicUnit=on
  Relational Operator1 : RelationalOperator  OutDataTypeStr=boolean  RndMeth=Simplest
  Repeating Sequence1 : simulink/Sources/Repeating Sequence  rep_seq_t=[0 Ts Ts*2]  rep_seq_y=[0 1 0]
  Repeating Sequence2 : simulink/Sources/Repeating Sequence  rep_seq_t=[0 Ts/2 Ts]  rep_seq_y=[0 1 0]
  Subsystem : Subsystem
  Subsystem2 : Subsystem
  Subsystem3 : Subsystem
  Switch : Switch  Criteria=u2 > Threshold  Threshold=1
  Terminator : Terminator
  Terminator1 : Terminator
  abc to dq0 : powerlib_meascontrol/Transformations/abc to dq0  Alignment=Aligned with phase A axis
  dq0 to Alpha-Beta-Zero : powerlib_meascontrol/Transformations/dq0 to Alpha-Beta-Zero  Alignment=Aligned with phase A axis
      settings: SourceProductBaseCode=PS
  G : Outport
  r : Outport  Port=2
  wires:
  Demux4/1 -> Subsystem/3(alpha), NTSV_7_nearest/1(Alpha)
  Demux/2 -> Subsystem3/2(q)
  Demux4/2 -> Subsystem/4(beta), NTSV_7_nearest/2(Beta)
  [theta_e] -> abc to dq0/2, dq0 to Alpha-Beta-Zero/2
  Demux/1 -> Subsystem3/1(d)
  Constant2/1 -> Add2/1
  Current/1 -> abc to dq0/1
  dU/1 -> Subsystem/5(dV)
  Subsystem2/1(Output) -> G/1
  abc to dq0/1 -> Demux/1
  Demux/3 -> Terminator/1
  Mux1/1 -> dq0 to Alpha-Beta-Zero/1
  Subsystem3/1(Ud) -> Subsystem/1(ud), Mux1/1
  Subsystem3/2(Uq) -> Subsystem/2(uq), Mux1/2
  Constant/1 -> Mux1/3
  dq0 to Alpha-Beta-Zero/1 -> Demux4/1
  Demux4/3 -> Terminator1/1
  NTSV_7_nearest/7(r) -> r/1
  Add2/1 -> Relational Operator1/2
  Relational Operator1/1 -> Subsystem2/1(Compare)
  NTSV_7_nearest/1(Ta1) -> Mux3/1
  NTSV_7_nearest/2(Ta2) -> Mux3/2
  NTSV_7_nearest/3(Tb1) -> Mux3/3
  NTSV_7_nearest/4(Tb2) -> Mux3/4
  NTSV_7_nearest/5(Tc1) -> Mux3/5
  NTSV_7_nearest/6(Tc2) -> Mux3/6
  Mux3/1 -> Add2/2
  Repeating Sequence2/1 -> Switch/1
  Repeating Sequence1/1 -> Switch/3
  Switch/1 -> Relational Operator1/1
  [state] -> Switch/2
  Subsystem/1(r) -> NTSV_7_nearest/3("r ")

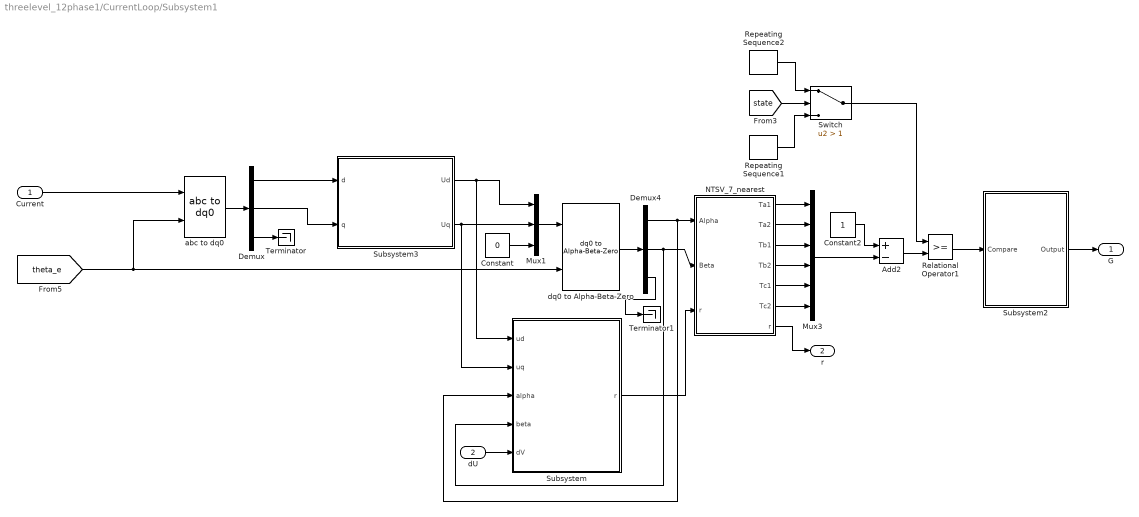
== system threelevel_12phase1/CurrentLoop/Subsystem1 ==
  Current : Inport
  dU : Inport  Port=2
  Add2 : Sum  Inputs=+-  AccumDataTypeStr=double  OutDataTypeStr=double
  Constant : Constant  Value=0
  Constant2 : Constant  OutDataTypeStr=double
  Demux : Demux  Outputs=3
  Demux4 : Demux  Outputs=3
  Mux1 : Mux  Inputs=3
  Mux3 : Mux  Inputs=6
  NTSV_7_nearest : MATLAB Function  TreatAsAtomicUnit=on
  Relational Operator1 : RelationalOperator  OutDataTypeStr=boolean  RndMeth=Simplest
  Repeating Sequence1 : simulink/Sources/Repeating Sequence  rep_seq_t=[0 Ts Ts*2]  rep_seq_y=[0 1 0]
  Repeating Sequence2 : simulink/Sources/Repeating Sequence  rep_seq_t=[0 Ts/2 Ts]  rep_seq_y=[0 1 0]
  Subsystem : Subsystem
  Subsystem2 : Subsystem
  Subsystem3 : Subsystem
  Switch : Switch  Criteria=u2 > Threshold  Threshold=1
  Terminator : Terminator
  Terminator1 : Terminator
  abc to dq0 : powerlib_meascontrol/Transformations/abc to dq0  Alignment=Aligned with phase A axis
  dq0 to Alpha-Beta-Zero : powerlib_meascontrol/Transformations/dq0 to Alpha-Beta-Zero  Alignment=Aligned with phase A axis
      settings: SourceProductBaseCode=PS
  G : Outport
  r : Outport  Port=2
  wires:
  Demux4/1 -> Subsystem/3(alpha), NTSV_7_nearest/1(Alpha)
  Demux/2 -> Subsystem3/2(q)
  Demux4/2 -> Subsystem/4(beta), NTSV_7_nearest/2(Beta)
  [theta_e] -> abc to dq0/2, dq0 to Alpha-Beta-Zero/2
  Demux/1 -> Subsystem3/1(d)
  Constant2/1 -> Add2/1
  Current/1 -> abc to dq0/1
  dU/1 -> Subsystem/5(dV)
  Subsystem2/1(Output) -> G/1
  abc to dq0/1 -> Demux/1
  Demux/3 -> Terminator/1
  Mux1/1 -> dq0 to Alpha-Beta-Zero/1
  Subsystem3/1(Ud) -> Subsystem/1(ud), Mux1/1
  Subsystem3/2(Uq) -> Subsystem/2(uq), Mux1/2
  Constant/1 -> Mux1/3
  dq0 to Alpha-Beta-Zero/1 -> Demux4/1
  Demux4/3 -> Terminator1/1
  NTSV_7_nearest/7(r) -> r/1
  Add2/1 -> Relational Operator1/2
  Relational Operator1/1 -> Subsystem2/1(Compare)
  NTSV_7_nearest/1(Ta1) -> Mux3/1
  NTSV_7_nearest/2(Ta2) -> Mux3/2
  NTSV_7_nearest/3(Tb1) -> Mux3/3
  NTSV_7_nearest/4(Tb2) -> Mux3/4
  NTSV_7_nearest/5(Tc1) -> Mux3/5
  NTSV_7_nearest/6(Tc2) -> Mux3/6
  Mux3/1 -> Add2/2
  Repeating Sequence2/1 -> Switch/1
  Repeating Sequence1/1 -> Switch/3
  Switch/1 -> Relational Operator1/1
  [state] -> Switch/2
  Subsystem/1(r) -> NTSV_7_nearest/3("r ")

== system threelevel_12phase1/CurrentLoop/Subsystem2 ==
  Current : Inport
  dU : Inport  Port=2
  Add2 : Sum  Inputs=+-  AccumDataTypeStr=double  OutDataTypeStr=double
  Constant : Constant  Value=0
  Constant2 : Constant  OutDataTypeStr=double
  Demux : Demux  Outputs=3
  Demux4 : Demux  Outputs=3
  Mux1 : Mux  Inputs=3
  Mux3 : Mux  Inputs=6
  NTSV_7_nearest : MATLAB Function  TreatAsAtomicUnit=on
  Relational Operator1 : RelationalOperator  OutDataTypeStr=boolean  RndMeth=Simplest
  Repeating Sequence1 : simulink/Sources/Repeating Sequence  rep_seq_t=[0 Ts Ts*2]  rep_seq_y=[0 1 0]
  Repeating Sequence2 : simulink/Sources/Repeating Sequence  rep_seq_t=[0 Ts/2 Ts]  rep_seq_y=[0 1 0]
  Subsystem : Subsystem
  Subsystem2 : Subsystem
  Subsystem3 : Subsystem
  Switch : Switch  Criteria=u2 > Threshold  Threshold=1
  Terminator : Terminator
  Terminator1 : Terminator
  abc to dq0 : powerlib_meascontrol/Transformations/abc to dq0  Alignment=Aligned with phase A axis
  dq0 to Alpha-Beta-Zero : powerlib_meascontrol/Transformations/dq0 to Alpha-Beta-Zero  Alignment=Aligned with phase A axis
      settings: SourceProductBaseCode=PS
  G : Outport
  r : Outport  Port=2
  wires:
  Demux4/1 -> Subsystem/3(alpha), NTSV_7_nearest/1(Alpha)
  Demux/2 -> Subsystem3/2(q)
  Demux4/2 -> Subsystem/4(beta), NTSV_7_nearest/2(Beta)
  [theta_e] -> abc to dq0/2, dq0 to Alpha-Beta-Zero/2
  Demux/1 -> Subsystem3/1(d)
  Constant2/1 -> Add2/1
  Current/1 -> abc to dq0/1
  dU/1 -> Subsystem/5(dV)
  Subsystem2/1(Output) -> G/1
  abc to dq0/1 -> Demux/1
  Demux/3 -> Terminator/1
  Mux1/1 -> dq0 to Alpha-Beta-Zero/1
  Subsystem3/1(Ud) -> Subsystem/1(ud), Mux1/1
  Subsystem3/2(Uq) -> Subsystem/2(uq), Mux1/2
  Constant/1 -> Mux1/3
  dq0 to Alpha-Beta-Zero/1 -> Demux4/1
  Demux4/3 -> Terminator1/1
  NTSV_7_nearest/7(r) -> r/1
  Add2/1 -> Relational Operator1/2
  Relational Operator1/1 -> Subsystem2/1(Compare)
  NTSV_7_nearest/1(Ta1) -> Mux3/1
  NTSV_7_nearest/2(Ta2) -> Mux3/2
  NTSV_7_nearest/3(Tb1) -> Mux3/3
  NTSV_7_nearest/4(Tb2) -> Mux3/4
  NTSV_7_nearest/5(Tc1) -> Mux3/5
  NTSV_7_nearest/6(Tc2) -> Mux3/6
  Mux3/1 -> Add2/2
  Repeating Sequence2/1 -> Switch/1
  Repeating Sequence1/1 -> Switch/3
  Switch/1 -> Relational Operator1/1
  [state] -> Switch/2
  Subsystem/1(r) -> NTSV_7_nearest/3("r ")

== system threelevel_12phase1/CurrentLoop/Subsystem3 ==
  Current : Inport
  dU : Inport  Port=2
  Add2 : Sum  Inputs=+-  AccumDataTypeStr=double  OutDataTypeStr=double
  Constant : Constant  Value=0
  Constant2 : Constant  OutDataTypeStr=double
  Demux : Demux  Outputs=3
  Demux4 : Demux  Outputs=3
  Mux1 : Mux  Inputs=3
  Mux3 : Mux  Inputs=6
  NTSV_7_nearest : MATLAB Function  TreatAsAtomicUnit=on
  Relational Operator1 : RelationalOperator  OutDataTypeStr=boolean  RndMeth=Simplest
  Repeating Sequence1 : simulink/Sources/Repeating Sequence  rep_seq_t=[0 Ts Ts*2]  rep_seq_y=[0 1 0]
  Repeating Sequence2 : simulink/Sources/Repeating Sequence  rep_seq_t=[0 Ts/2 Ts]  rep_seq_y=[0 1 0]
  Subsystem : Subsystem
  Subsystem2 : Subsystem
  Subsystem3 : Subsystem
  Switch : Switch  Criteria=u2 > Threshold  Threshold=1
  Terminator : Terminator
  Terminator1 : Terminator
  abc to dq0 : powerlib_meascontrol/Transformations/abc to dq0  Alignment=Aligned with phase A axis
  dq0 to Alpha-Beta-Zero : powerlib_meascontrol/Transformations/dq0 to Alpha-Beta-Zero  Alignment=Aligned with phase A axis
      settings: SourceProductBaseCode=PS
  G : Outport
  r : Outport  Port=2
  wires:
  Demux4/1 -> Subsystem/3(alpha), NTSV_7_nearest/1(Alpha)
  Demux/2 -> Subsystem3/2(q)
  Demux4/2 -> Subsystem/4(beta), NTSV_7_nearest/2(Beta)
  [theta_e] -> abc to dq0/2, dq0 to Alpha-Beta-Zero/2
  Demux/1 -> Subsystem3/1(d)
  Constant2/1 -> Add2/1
  Current/1 -> abc to dq0/1
  dU/1 -> Subsystem/5(dV)
  Subsystem2/1(Output) -> G/1
  abc to dq0/1 -> Demux/1
  Demux/3 -> Terminator/1
  Mux1/1 -> dq0 to Alpha-Beta-Zero/1
  Subsystem3/1(Ud) -> Subsystem/1(ud), Mux1/1
  Subsystem3/2(Uq) -> Subsystem/2(uq), Mux1/2
  Constant/1 -> Mux1/3
  dq0 to Alpha-Beta-Zero/1 -> Demux4/1
  Demux4/3 -> Terminator1/1
  NTSV_7_nearest/7(r) -> r/1
  Add2/1 -> Relational Operator1/2
  Relational Operator1/1 -> Subsystem2/1(Compare)
  NTSV_7_nearest/1(Ta1) -> Mux3/1
  NTSV_7_nearest/2(Ta2) -> Mux3/2
  NTSV_7_nearest/3(Tb1) -> Mux3/3
  NTSV_7_nearest/4(Tb2) -> Mux3/4
  NTSV_7_nearest/5(Tc1) -> Mux3/5
  NTSV_7_nearest/6(Tc2) -> Mux3/6
  Mux3/1 -> Add2/2
  Repeating Sequence2/1 -> Switch/1
  Repeating Sequence1/1 -> Switch/3
  Switch/1 -> Relational Operator1/1
  [state] -> Switch/2
  Subsystem/1(r) -> NTSV_7_nearest/3("r ")

== system threelevel_12phase1/Mech/生成转速波动 ==
  Add : Sum
  Add2 : Sum  Inputs=-+
  Product3 : Product
  Repeating Sequence : simulink/Sources/Repeating Sequence  rep_seq_t=[0 0.1]  rep_seq_y=[0 1]
  Uniform Random Number : UniformRandomNumber  Minimum=0.9  Maximum=1.1  Seed=123  SampleTime=0.1
  Unit Delay : UnitDelay  SampleTime=-1  HasFrameUpgradeWarning=on
  Out1 : Outport
  wires:
  Product3/1 -> Add/2
  Repeating Sequence/1 -> Product3/2
  Uniform Random Number/1 -> Add2/2, Unit Delay/1
  Add2/1 -> Product3/1
  Unit Delay/1 -> Add2/1, Add/1
  Add/1 -> Out1/1

== system threelevel_12phase1/CurrentLoop/Subsystem/Subsystem ==
  ud : Inport
  uq : Inport  Port=2
  alpha : Inport  Port=3
  beta : Inport  Port=4
  dV : Inport  Port=5
  Atan2 : Trigonometry  Operator=atan2
  Constant : Constant
  Constant1 : Constant  Value=VDC
  Constant7 : Constant
  Divide : Product  Inputs=*/
  First_Order2 : Subsystem
  Gain : Gain  Gain=10
  PID Controller1 : slpidlib/PID Controller  Controller=PI  Form=Parallel  TimeDomain=Discrete-time  UseExternalTs=off  SampleTime=Ts  IntegratorMethod=Forward Euler  FilterMethod=Forward Euler  ControllerParametersSource=external  P=1/VDC  I=1/VDC  D=0  UseFilter=on  N=100  TunerSelectOption=Transfer Function Based (PID Tuner App)  InitialConditionSource=internal  InitialConditionForIntegrator=0  InitialConditionForFilter=0  DifferentiatorICPrevScaledInput=0  ExternalReset=none  TrackingMode=off  Kt=1  LimitOutput=on  SatLimitsSource=internal  UpperSaturationLimit=1  LowerSaturationLimit=-1  LinearizeAsGain=off  AntiWindupMode=none  Kb=1  POutMin=[]  POutMax=[]  IOutMin=[]  IOutMax=[]  DOutMin=[]  DOutMax=[]  NOutMin=[]  NOutMax=[]  SumOutMin=[]  SumOutMax=[]  SaturationOutMin=[]  SaturationOutMax=[]  PParamMin=[]  PParamMax=[]  IParamMin=[]  IParamMax=[]  DParamMin=[]  DParamMax=[]  NParamMin=[]  NParamMax=[]  KbParamMin=[]  KbParamMax=[]  KtParamMin=[]  KtParamMax=[]  KbOutMin=[]  KbOutMax=[]  KtOutMin=[]  KtOutMax=[]  IntegratorOutMin=[]  IntegratorOutMax=[]  FilterOutMin=[]  FilterOutMax=[]  SumI1OutMin=[]  SumI1OutMax=[]  SumI2OutMin=[]  SumI2OutMax=[]  SumI3OutMin=[]  SumI3OutMax=[]  SumI4OutMin=[]  SumI4OutMax=[]  SumDOutMin=[]  SumDOutMax=[]  DifferentiatorOutMin=[]  DifferentiatorOutMax=[]  FilterDiffOutCoefMin=[]  FilterDiffOutCoefMax=[]  ReciprocalOutMin=[]  ReciprocalOutMax=[]  SumDenOutMin=[]  SumDenOutMax=[]  SumNumOutMin=[]  SumNumOutMax=[]  DivideOutMin=[]  DivideOutMax=[]  UdiffTsProdOutMin=[]  UdiffTsProdOutMax=[]  NTsProdOutMin=[]  NTsProdOutMax=[]  UintegralTsProdOutMin=[]  UintegralTsProdOutMax=[]  UngainTsProdOutMin=[]  UngainTsProdOutMax=[]  IntegratorContinuousStateAttributes=''  IntegratorStateMustResolveToSignalObject=off  IntegratorRTWStateStorageClass=Auto  FilterContinuousStateAttributes=''  FilterStateMustResolveToSignalObject=off  FilterRTWStateStorageClass=Auto  ParallelPVariant=ExternalParameters  IdealPVariant=Disabled  IVariant=ExternalParameters  DVariant=Disabled  IntegratorVariant=Discrete  SatVariant=Enabled  AWVariant=Passthrough  PCopyVariant=Disabled  TRVariant=Disabled  FdbkBlocksVariant=Forward  IdealPFdbkVariant=Disabled  SatFdbkVariant=Disabled  DerivativeFilterVariant=Disabled  NVariant=Disabled  NCopyVariant=Disabled_SignalSpec  FilterICVariant=Disabled  IntegratorICVariant=InternalICs  ExternalResetVariant=Disabled  TRSumVariant=Passthrough  SumFdbkVariant=Disabled  SumVariant=Sum_PI  TsampFilterVariant=InternalTs  TsampNgainVariant=Passthrough  TsampIntegralVariant=Passthrough  ExternalSaturationOutDataTypeStr=Inherit: Same as second input
  Product1 : Product
  Saturation1 : Saturate  UpperLimit=1  LowerLimit=-1
  propose method1 : MATLAB Function  TreatAsAtomicUnit=on
  针对负载波动的P增量 : Subsystem  Commented=on
  r : Outport
  wires:
  Divide/1 -> Product1/1, Gain/1
  Constant1/1 -> Divide/2
  Constant7/1 -> Divide/1
  alpha/1 -> propose method1/2(alpha)
  uq/1 -> Atan2/2
  beta/1 -> propose method1/3(beta)
  propose method1/1(r) -> Saturation1/1
  Atan2/1 -> First_Order2/1(In1)
  ud/1 -> Atan2/1
  dV/1 -> PID Controller1/1
  Constant/1 -> Product1/2
  Gain/1 -> PID Controller1/3
  Product1/1 -> PID Controller1/2
  First_Order2/1(ADC_temp) -> propose method1/4(phi)
  Saturation1/1 -> r/1
  PID Controller1/1 -> propose method1/1(PI)

== system threelevel_12phase1/CurrentLoop/Subsystem/Subsystem2 ==
  Compare : Inport
  AND13 : Logic  AllPortsSameDT=off  OutDataTypeStr=boolean
  AND14 : Logic  AllPortsSameDT=off  OutDataTypeStr=boolean
  Delay13 : Delay  DelayLength=Ts_Dead/Ts_FEA
  Demux : Demux  Outputs=6
  Demux1 : Demux  Outputs=6
  Mux : Mux  Inputs=12
  NOT6 : Logic  Operator=NOT  AllPortsSameDT=off  OutDataTypeStr=boolean
  NOT7 : Logic  Operator=NOT  AllPortsSameDT=off  OutDataTypeStr=boolean
  Output : Outport
  wires:
  Mux/1 -> Output/1
  Compare/1 -> Delay13/1, NOT6/1, AND13/1
  Delay13/1 -> NOT7/1, AND13/2
  NOT7/1 -> AND14/1
  NOT6/1 -> AND14/2
  AND13/1 -> Demux/1
  AND14/1 -> Demux1/1
  Demux/1 -> Mux/1
  Demux/2 -> Mux/2
  Demux/3 -> Mux/5
  Demux/4 -> Mux/6
  Demux/5 -> Mux/9
  Demux/6 -> Mux/10
  Demux1/1 -> Mux/3
  Demux1/2 -> Mux/4
  Demux1/3 -> Mux/7
  Demux1/4 -> Mux/8
  Demux1/5 -> Mux/11
  Demux1/6 -> Mux/12

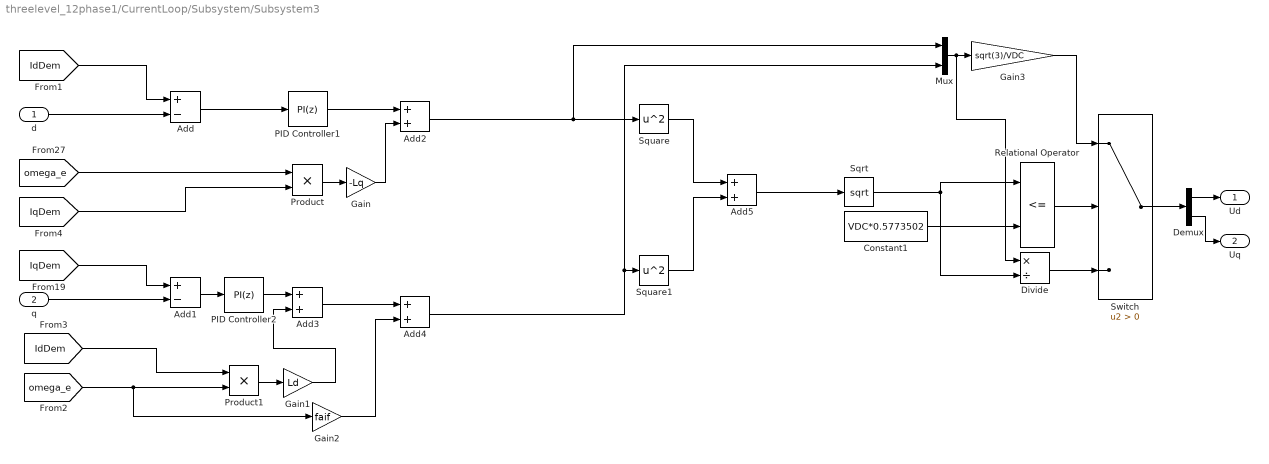
== system threelevel_12phase1/CurrentLoop/Subsystem/Subsystem3 ==
  d : Inport
  q : Inport  Port=2
  Add : Sum  Inputs=+-
  Add1 : Sum  Inputs=+-
  Add{2..5} (4 alike) : Sum
  Constant1 : Constant  Value=VDC*0.5773502
  Demux : Demux  Outputs=2
  Divide : Product  Inputs=*/
  Gain : Gain  Gain=-Lq
  Gain1 : Gain  Gain=Ld
  Gain2 : Gain  Gain=faif
  Gain3 : Gain  Gain=sqrt(3)/VDC
  Mux : Mux  Inputs=2
  PID Controller1 : slpidlib/PID Controller  Controller=PI  Form=Parallel  TimeDomain=Discrete-time  UseExternalTs=off  SampleTime=Ts  IntegratorMethod=Forward Euler  FilterMethod=Forward Euler  ControllerParametersSource=internal  P=ws*2*pi*Ld  I=ws*2*pi*Rs  D=0  UseFilter=on  N=100  TunerSelectOption=Transfer Function Based (PID Tuner App)  InitialConditionSource=internal  InitialConditionForIntegrator=0  InitialConditionForFilter=0  DifferentiatorICPrevScaledInput=0  ExternalReset=none  TrackingMode=off  Kt=1  LimitOutput=off  SatLimitsSource=internal  UpperSaturationLimit=inf  LowerSaturationLimit=-inf  LinearizeAsGain=on  AntiWindupMode=none  Kb=1  POutMin=[]  POutMax=[]  IOutMin=[]  IOutMax=[]  DOutMin=[]  DOutMax=[]  NOutMin=[]  NOutMax=[]  SumOutMin=[]  SumOutMax=[]  SaturationOutMin=[]  SaturationOutMax=[]  PParamMin=[]  PParamMax=[]  IParamMin=[]  IParamMax=[]  DParamMin=[]  DParamMax=[]  NParamMin=[]  NParamMax=[]  KbParamMin=[]  KbParamMax=[]  KtParamMin=[]  KtParamMax=[]  KbOutMin=[]  KbOutMax=[]  KtOutMin=[]  KtOutMax=[]  IntegratorOutMin=[]  IntegratorOutMax=[]  FilterOutMin=[]  FilterOutMax=[]  SumI1OutMin=[]  SumI1OutMax=[]  SumI2OutMin=[]  SumI2OutMax=[]  SumI3OutMin=[]  SumI3OutMax=[]  SumI4OutMin=[]  SumI4OutMax=[]  SumDOutMin=[]  SumDOutMax=[]  DifferentiatorOutMin=[]  DifferentiatorOutMax=[]  FilterDiffOutCoefMin=[]  FilterDiffOutCoefMax=[]  ReciprocalOutMin=[]  ReciprocalOutMax=[]  SumDenOutMin=[]  SumDenOutMax=[]  SumNumOutMin=[]  SumNumOutMax=[]  DivideOutMin=[]  DivideOutMax=[]  UdiffTsProdOutMin=[]  UdiffTsProdOutMax=[]  NTsProdOutMin=[]  NTsProdOutMax=[]  UintegralTsProdOutMin=[]  UintegralTsProdOutMax=[]  UngainTsProdOutMin=[]  UngainTsProdOutMax=[]  IntegratorContinuousStateAttributes=''  IntegratorStateMustResolveToSignalObject=off  IntegratorRTWStateStorageClass=Auto  FilterContinuousStateAttributes=''  FilterStateMustResolveToSignalObject=off  FilterRTWStateStorageClass=Auto  ParallelPVariant=InternalParameters  IdealPVariant=Disabled  IVariant=InternalParameters  DVariant=Disabled  IntegratorVariant=Discrete  SatVariant=Disabled  AWVariant=Passthrough  PCopyVariant=Disabled  TRVariant=Disabled  FdbkBlocksVariant=Forward  IdealPFdbkVariant=Disabled  SatFdbkVariant=Disabled  DerivativeFilterVariant=Disabled  NVariant=Disabled  NCopyVariant=Disabled_SignalSpec  FilterICVariant=Disabled  IntegratorICVariant=InternalICs  ExternalResetVariant=Disabled  TRSumVariant=Passthrough  SumFdbkVariant=Disabled  SumVariant=Sum_PI  TsampFilterVariant=InternalTs  TsampNgainVariant=Passthrough  TsampIntegralVariant=Passthrough  ExternalSaturationOutDataTypeStr=Inherit: Same as second input
  PID Controller2 : slpidlib/PID Controller  Controller=PI  Form=Parallel  TimeDomain=Discrete-time  UseExternalTs=off  SampleTime=Ts  IntegratorMethod=Forward Euler  FilterMethod=Forward Euler  ControllerParametersSource=internal  P=ws*2*pi*Lq  I=ws*2*pi*Rs  D=0  UseFilter=on  N=100  TunerSelectOption=Transfer Function Based (PID Tuner App)  InitialConditionSource=internal  InitialConditionForIntegrator=0  InitialConditionForFilter=0  DifferentiatorICPrevScaledInput=0  ExternalReset=none  TrackingMode=off  Kt=1  LimitOutput=off  SatLimitsSource=internal  UpperSaturationLimit=inf  LowerSaturationLimit=-inf  LinearizeAsGain=on  AntiWindupMode=none  Kb=1  POutMin=[]  POutMax=[]  IOutMin=[]  IOutMax=[]  DOutMin=[]  DOutMax=[]  NOutMin=[]  NOutMax=[]  SumOutMin=[]  SumOutMax=[]  SaturationOutMin=[]  SaturationOutMax=[]  PParamMin=[]  PParamMax=[]  IParamMin=[]  IParamMax=[]  DParamMin=[]  DParamMax=[]  NParamMin=[]  NParamMax=[]  KbParamMin=[]  KbParamMax=[]  KtParamMin=[]  KtParamMax=[]  KbOutMin=[]  KbOutMax=[]  KtOutMin=[]  KtOutMax=[]  IntegratorOutMin=[]  IntegratorOutMax=[]  FilterOutMin=[]  FilterOutMax=[]  SumI1OutMin=[]  SumI1OutMax=[]  SumI2OutMin=[]  SumI2OutMax=[]  SumI3OutMin=[]  SumI3OutMax=[]  SumI4OutMin=[]  SumI4OutMax=[]  SumDOutMin=[]  SumDOutMax=[]  DifferentiatorOutMin=[]  DifferentiatorOutMax=[]  FilterDiffOutCoefMin=[]  FilterDiffOutCoefMax=[]  ReciprocalOutMin=[]  ReciprocalOutMax=[]  SumDenOutMin=[]  SumDenOutMax=[]  SumNumOutMin=[]  SumNumOutMax=[]  DivideOutMin=[]  DivideOutMax=[]  UdiffTsProdOutMin=[]  UdiffTsProdOutMax=[]  NTsProdOutMin=[]  NTsProdOutMax=[]  UintegralTsProdOutMin=[]  UintegralTsProdOutMax=[]  UngainTsProdOutMin=[]  UngainTsProdOutMax=[]  IntegratorContinuousStateAttributes=''  IntegratorStateMustResolveToSignalObject=off  IntegratorRTWStateStorageClass=Auto  FilterContinuousStateAttributes=''  FilterStateMustResolveToSignalObject=off  FilterRTWStateStorageClass=Auto  ParallelPVariant=InternalParameters  IdealPVariant=Disabled  IVariant=InternalParameters  DVariant=Disabled  IntegratorVariant=Discrete  SatVariant=Disabled  AWVariant=Passthrough  PCopyVariant=Disabled  TRVariant=Disabled  FdbkBlocksVariant=Forward  IdealPFdbkVariant=Disabled  SatFdbkVariant=Disabled  DerivativeFilterVariant=Disabled  NVariant=Disabled  NCopyVariant=Disabled_SignalSpec  FilterICVariant=Disabled  IntegratorICVariant=InternalICs  ExternalResetVariant=Disabled  TRSumVariant=Passthrough  SumFdbkVariant=Disabled  SumVariant=Sum_PI  TsampFilterVariant=InternalTs  TsampNgainVariant=Passthrough  TsampIntegralVariant=Passthrough  ExternalSaturationOutDataTypeStr=Inherit: Same as second input
  Product : Product
  Product1 : Product
  Relational Operator : RelationalOperator  Operator=<=  OutDataTypeStr=boolean  RndMeth=Simplest
  Sqrt : Sqrt  SaturateOnIntegerOverflow=on
  Square : Math  Operator=square  SaturateOnIntegerOverflow=on
  Square1 : Math  Operator=square  SaturateOnIntegerOverflow=on
  Switch : Switch  Criteria=u2 > Threshold
  Ud : Outport
  Uq : Outport  Port=2
  wires:
  d/1 -> Add/2
  q/1 -> Add1/2
  [IqDem] -> Add1/1
  Add/1 -> PID Controller1/1
  Add1/1 -> PID Controller2/1
  PID Controller1/1 -> Add2/1
  [omega_e] -> Product/1
  Product/1 -> Gain/1
  Gain/1 -> Add2/2
  PID Controller2/1 -> Add3/1
  Product1/1 -> Gain1/1
  Gain1/1 -> Add3/2
  Add3/1 -> Add4/1
  Gain2/1 -> Add4/2
  [omega_e] -> Gain2/1, Product1/2
  Add2/1 -> Square/1, Mux/1
  Add4/1 -> Mux/2, Square1/1
  Square/1 -> Add5/1
  Square1/1 -> Add5/2
  Sqrt/1 -> Relational Operator/1, Divide/2
  Constant1/1 -> Relational Operator/2
  Relational Operator/1 -> Switch/2
  Switch/1 -> Demux/1
  Demux/1 -> Ud/1
  Demux/2 -> Uq/1
  Mux/1 -> Divide/1, Gain3/1
  Gain3/1 -> Switch/1
  Divide/1 -> Switch/3
  [IdDem] -> Add/1
  [IdDem] -> Product1/1
  [IqDem] -> Product/2
  Add5/1 -> Sqrt/1
